simulink model "massSpringDamper"  (R2013b)
settings: Solver=ode45  StartTime=0.0  StopTime=experimentStopTime  MaxStep=dt  RelTol=1e-3
InitFcn:
  | massSpringDamper_init;
StopFcn:
  | massSpringDamper_stop;
values from neighbouring files (symbols this model uses):
  c = 0.2    [massSpringDamper_init.m]
  experimentStopTime = 60    [massSpringDamper_init.m]
  k = 0.8    [massSpringDamper_init.m]
  m = 1    [massSpringDamper_init.m]
libraries: simulink x1
settings Model: Creator=LabUser  LastModifiedBy=jaustin
settings OptimizationCC: ExpressionDepthLimit=2147483647
settings DebuggingCC: StateNameClashWarn=warning

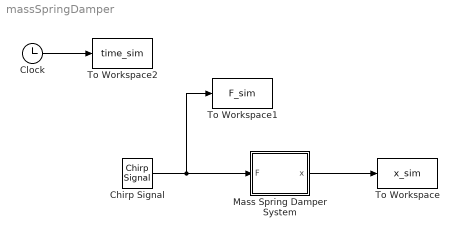
== system massSpringDamper ==
  Chirp Signal : simulink/Sources/Chirp Signal  f1=wmin  T=experimentStopTime  f2=wmax
  Clock : Clock
  Mass Spring Damper System : Subsystem
  To Workspace : ToWorkspace  VariableName=x_sim  SampleTime=-1
  To Workspace1 : ToWorkspace  VariableName=F_sim  SampleTime=-1
  To Workspace2 : ToWorkspace  VariableName=time_sim  SampleTime=-1
  wires:
  Mass Spring Damper System/1(x) -> To Workspace/1
  Chirp Signal/1 -> To Workspace1/1, Mass Spring Damper System/1(F)
  Clock/1 -> To Workspace2/1

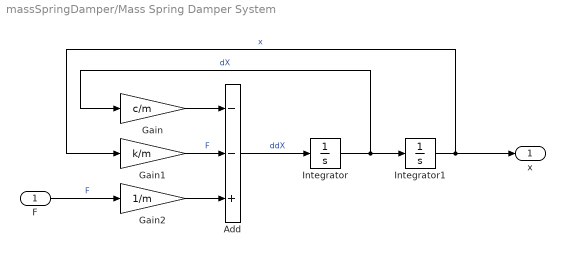
== system massSpringDamper/Mass Spring Damper System ==
  F : Inport
  Add : Sum  Inputs=--+
  Gain : Gain  Gain=c/m
  Gain1 : Gain  Gain=k/m
  Gain2 : Gain  Gain=1/m
  Integrator : Integrator
  Integrator1 : Integrator
  x : Outport
  wires:
  Add/1 -> Integrator/1  "ddX"
  F/1 -> Gain2/1  "F"
  Gain1/1 -> Add/2  "F"
  Gain/1 -> Add/1
  Integrator/1 -> Gain/1, Integrator1/1  "dX"
  Integrator1/1 -> x/1, Gain1/1  "x"
  Gain2/1 -> Add/3
